simulink subsystem "torqueCommand"  (R2022b)
settings: Solver=VariableStepAuto  StartTime=0.0  StopTime=10.0  RelTol=1e-3
libraries: Raptor_lib x1, torqueCommand_lib x1
settings Model: Creator=serga  LastModifiedBy=serga

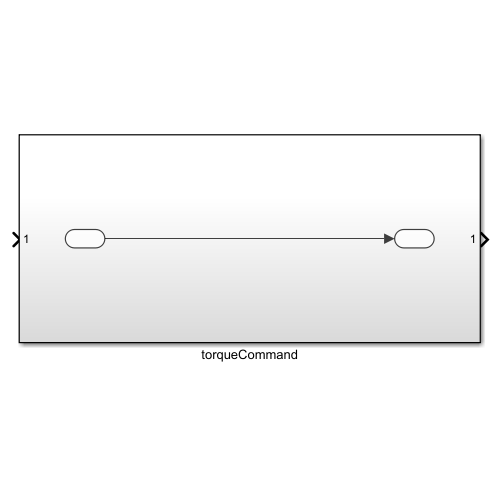
[thumbnail: Simulink's stored preview of the top-level diagram]
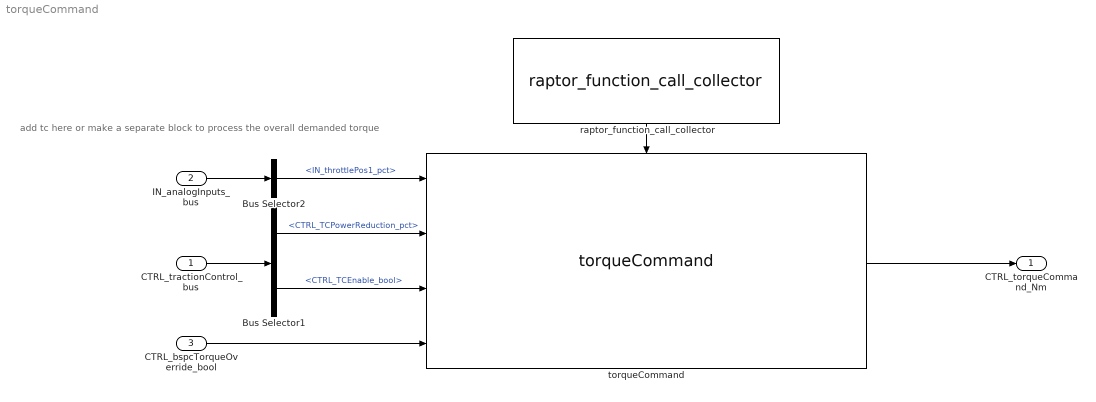
== system torqueCommand ==
  note: add tc here or make a separate block to process the overall demanded torque
  CTRL_tractionControl_bus : Inport
  IN_analogInputs_bus : Inport  Port=2
  CTRL_bspcTorqueOverride_bool : Inport  Port=3
  Bus Selector1 : BusSelector  OutputSignals=CTRL_TCPowerReduction_pct,CTRL_TCEnable_bool
  Bus Selector2 : BusSelector  OutputSignals=IN_throttle_bus.IN_throttle1_bus.IN_throttlePos1_pct
  raptor_function_call_collector : Raptor_lib/Triggers/raptor_function_call_collector  count=5
      settings: SourceProductName=Raptor
  torqueCommand : torqueCommand_lib/torqueCommand  SystemSampleTime=-1  VariantActivationTime=update diagram  Latency=0  AutoFrameSizeCalculation=off
  CTRL_torqueCommand_Nm : Outport
  wires:
  raptor_function_call_collector/1 -> torqueCommand/Trigger
  torqueCommand/1 -> CTRL_torqueCommand_Nm/1
  CTRL_tractionControl_bus/1 -> Bus Selector1/1
  Bus Selector1/1 -> torqueCommand/2  "<CTRL_TCPowerReduction_pct>"
  Bus Selector1/2 -> torqueCommand/3  "<CTRL_TCEnable_bool>"
  IN_analogInputs_bus/1 -> Bus Selector2/1
  Bus Selector2/1 -> torqueCommand/1  "<IN_throttlePos1_pct>"
  CTRL_bspcTorqueOverride_bool/1 -> torqueCommand/4
